simulink model "Webcam_motor_test3"  (Simulink 7.3)
settings: Solver=FixedStepDiscrete  StartTime=0.0  StopTime=inf  MaxStep=0.2  RelTol=1e-3
settings Model: Creator=gclayton  LastModifiedBy=wildcat
settings DebuggingCC: InheritedTsInSrcMsg=none
settings RTWCC: SystemTargetFile=rlnx.tlc  GenCodeOnly=on  TemplateMakefile=rlnx_ubuntu.tmf  Description=Linux Real-Time Target  ProcessScript=rlnx_make_rtw_hook
settings RTWCC: CustomInclude=|
  | /usr/local/include/opencv/
  | /usr/local/include/
settings CodeAppCC: GenerateComments=off  SimulinkBlockComments=off
settings STFCustomTargetCC: ModelReferenceCompliant=off  MatFileLogging=on  SystemTargetFile=rlnx.tlc
settings GRTTargetCC: ModelReferenceCompliant=off  ParMdlRefBuildCompliant=off  CompOptLevelCompliant=off
settings CustomProperty: DataType=string  Value=-lm -ldl /usr/local/lib/libopencv_highgui.so.2.4
settings EnumStrPairs: String=PC

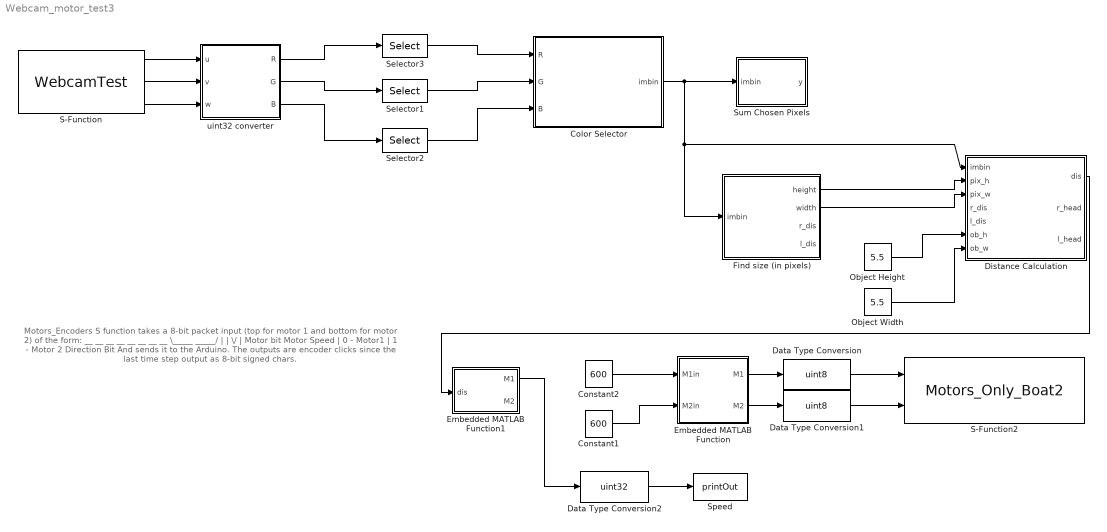
== system Webcam_motor_test3 ==
  note: Motors_Encoders S function takes a 8-bit packet input
      | (top for motor 1 and bottom for motor 2) of the form:
      |
      |          __ __ __ __ __ __ __ __
      |         \_____   _____/   |    |
      |                               \/              |  Motor bit
      |                          Motor Speed    |   0 - Motor1
      |                                                    |   1 - Motor 2
      |                                Direction Bit
      |
      | And sends it to the Arduino.  The outputs are encoder clicks
      | since the last time step output as 8-bit signed chars.
  Color Selector : Stateflow chart  TreatAsAtomicUnit=on
  Constant1 : Constant  Value=600
  Constant2 : Constant  Value=600
  Data Type Conversion : DataTypeConversion  OutDataTypeMode=uint8  OutDataTypeStr=uint8
  Data Type Conversion1 : DataTypeConversion  OutDataTypeMode=uint8  OutDataTypeStr=uint8
  Data Type Conversion2 : DataTypeConversion  OutDataTypeMode=uint32  OutDataTypeStr=uint32
  Distance Calculation : Stateflow chart  TreatAsAtomicUnit=on
  Embedded MATLAB Function : Stateflow chart  TreatAsAtomicUnit=on
  Embedded MATLAB Function1 : Stateflow chart
  Find size (in pixels) : Stateflow chart  TreatAsAtomicUnit=on
  Object Height : Constant  Value=5.5
  Object Width : Constant  Value=5.5
  S-Function : S-Function  FunctionName=WebcamTest  EnableBusSupport=off
  S-Function2 : S-Function  FunctionName=Motors_Only_Boat2  EnableBusSupport=off
  Selector1 : Selector  NumberOfDimensions=2  InputPortWidth=3  IndexOptions=Starting index (dialog),Starting index (dialog)  Indices=70,1  OutputSizes=340,640
  Selector2 : Selector  NumberOfDimensions=2  InputPortWidth=3  IndexOptions=Starting index (dialog),Starting index (dialog)  Indices=70,1  OutputSizes=340,640
  Selector3 : Selector  NumberOfDimensions=2  InputPortWidth=3  IndexOptions=Starting index (dialog),Starting index (dialog)  Indices=70,1  OutputSizes=340,640
  Speed : S-Function  FunctionName=printOut  EnableBusSupport=off
  Sum Chosen Pixels : Stateflow chart  TreatAsAtomicUnit=on
  uint32 converter : Stateflow chart  TreatAsAtomicUnit=on
  wires:
  S-Function/1 -> uint32 converter/1(u)
  S-Function/2 -> uint32 converter/2(v)
  S-Function/3 -> uint32 converter/3(w)
  Color Selector/1(imbin) -> Sum Chosen Pixels/1(imbin), Find size (in pixels)/1(imbin), Distance Calculation/1(imbin)
  Embedded MATLAB Function/1(M1) -> Data Type Conversion/1
  Embedded MATLAB Function/2(M2) -> Data Type Conversion1/1
  Data Type Conversion/1 -> S-Function2/1
  Data Type Conversion1/1 -> S-Function2/2
  Find size (in pixels)/1(height) -> Distance Calculation/2(pix_h)
  Find size (in pixels)/2(width) -> Distance Calculation/3(pix_w)
  Object Height/1 -> Distance Calculation/6(ob_h)
  Object Width/1 -> Distance Calculation/7(ob_w)
  uint32 converter/3(B) -> Selector2/1
  uint32 converter/2(G) -> Selector1/1
  uint32 converter/1(R) -> Selector3/1
  Selector3/1 -> Color Selector/1(R)
  Selector1/1 -> Color Selector/2(G)
  Selector2/1 -> Color Selector/3(B)
  Distance Calculation/1(dis) -> Embedded MATLAB Function1/1(dis)
  Constant2/1 -> Embedded MATLAB Function/1(M1in)
  Embedded MATLAB Function1/1(M1) -> Data Type Conversion2/1
  Data Type Conversion2/1 -> Speed/1
  Constant1/1 -> Embedded MATLAB Function/2(M2in)

== matlab function uint32 converter ==
  data: u input double; R output double; v input double; w input double; G output double; B output double
function [R,G,B]= fcn(u,v,w)

R = uint32(u);
G = uint32(v);
B = uint32(w);

== matlab function Sum Chosen Pixels ==
  data: imbin input double; y output double
function y = fcn(imbin)
%#eml

imsize = size(imbin);
red_pix = 0;

for (imh = 1:imsize(1,1));
    for (iml = 1:imsize(1,2));
        im_pix = imbin(imh,iml);     
        if (im_pix == 1)
           red_pix = red_pix+1;
        end
    end
end

y = uint32(red_pix);

== matlab function Color Selector ==
  data: R input double; G input double; B input double; imbin output double
function imbin  = color_selection(R,G,B)

imsize = size(R);
imsize = size(G);
imsize = size(B);

R1 = zeros(imsize);
G1 = zeros(imsize);
B1 = zeros(imsize);
imbin = zeros(imsize);

for (imh = 1:imsize(1,1));
    for (iml = 1:imsize(1,2));
        imR = R(imh,iml);
        imG = G(imh,iml);
        imB = B(imh,iml);
        if (imR >= 170) && (imR <= 255) && (imG >= 15) && (imG <= 70) && (imB >= 70) && (imB <= 130)
            R1(imh,iml) = 255;
            G1(imh,iml) = 255;
            B1(imh,iml) = 255;
            imbin(imh,iml) = 1;
        end
    end
end

== matlab function Find size (in pixels) ==
  data: imbin input double; height output double; width output double; r_dis output double; l_dis output double
function [height,width,r_dis,l_dis] = hw_find(imbin)

imsize=size(imbin);

height = 0;
width = 0;
height_sum = 0;
width_sum = 0;
marker = 0;
obstart = 0;

for (imh = 1:imsize(1,1));
    width_sum = 0;
    for (iml = 1:imsize(1,2));
        imloc = imbin(imh,iml);
        if (imloc == 1)
            width_sum=width_sum+1;
        end
    end
    if (width_sum >= 6)
        height = height+1;
    end
end



for (iml = 1:imsize(1,2));
    height_sum = 0;
    for (imh = 1:imsize(1,1));
        imloc = imbin(imh,iml);
        if (imloc == 1)
            height_sum=height_sum+1;
        end
    end
    if (height_sum >= 6)
        width = width+1;
        if (marker == 0)
            marker = 1;
            obstart = iml;
        end
    end
end

obend = obstart + width;

r_dis = obstart;
l_dis = imsize(1,2) - obend;

== matlab function Embedded MATLAB Function ==
  data: M1in input double; M1 output double; M2in input double; M2 output double
function [M1, M2] = MotorPackets(M1in, M2in)
%#eml

M1 = 0;
M2 = 1;

if M1in <= 0
    M1 = M1+2;
end

if M2in <= 0
    M2 = M2+2;
end

M1 = M1 + round(abs(M1in)*0.1)*4;
M2 = M2 + round(abs(M2in)*0.1)*4;

== matlab function Distance Calculation ==
  data: imbin input double; pix_h input double; dis output double; pix_w input double; r_dis input double; l_dis input double; ob_h input double; ob_w input double; r_head output double; l_head output double
function [dis,r_head,l_head] = find_dis(imbin,pix_h,pix_w,r_dis,l_dis,ob_h,ob_w)

%1.4=2*tan(44.443*pi/360)*dis*height1/480;
%ob_w=2*tan(57.154*pi/360)*dis*width1/640;

imsize = size(imbin);

dis1 = (ob_h*imsize(1,1))/(2*tan(44.443*pi/360)*pix_h);

dis2 = (ob_w*imsize(1,2))/(2*tan(57.154*pi/360)*pix_w);

r_head = (ob_w*imsize(1,2))/(2*tan(57.153*pi/360)*pix_w)*(r_dis/pix_w);

l_head = (ob_w*imsize(1,2))/(2*tan(57.153*pi/360)*pix_w)*(l_dis/pix_w);

dis=(dis1+3*dis2)/4;

== matlab function Embedded MATLAB Function1 ==
  data: dis input double; M1 output double; M2 output double
function [M1,M2]= fcn(dis)

%Sample speed
M1 = 620-5*dis;
M2 = 620-5*dis;


%Prevent rpm of M1 and M2 from going above 620 or below -620
if (M1 >= 620)
    M1 = 620;
elseif (M1<= -620)
    M2 = -620;
else
    M1 = M1;
end


if (M2 >= 620)
    M2 = 620;
elseif (M2<= -620)
    M2 = -620;
else
    M2 = M2;
end
